simulink model "DCMotorSystem"  (R2018b)
settings: Solver=FixedStepAuto  StartTime=0.0  StopTime=50  FixedStep=10^-5  RelTol=1e-3
undefined symbols (not defined in the file or in its folder): Kd, Kp
settings Model: Creator=Seko  LastModifiedBy=Seko

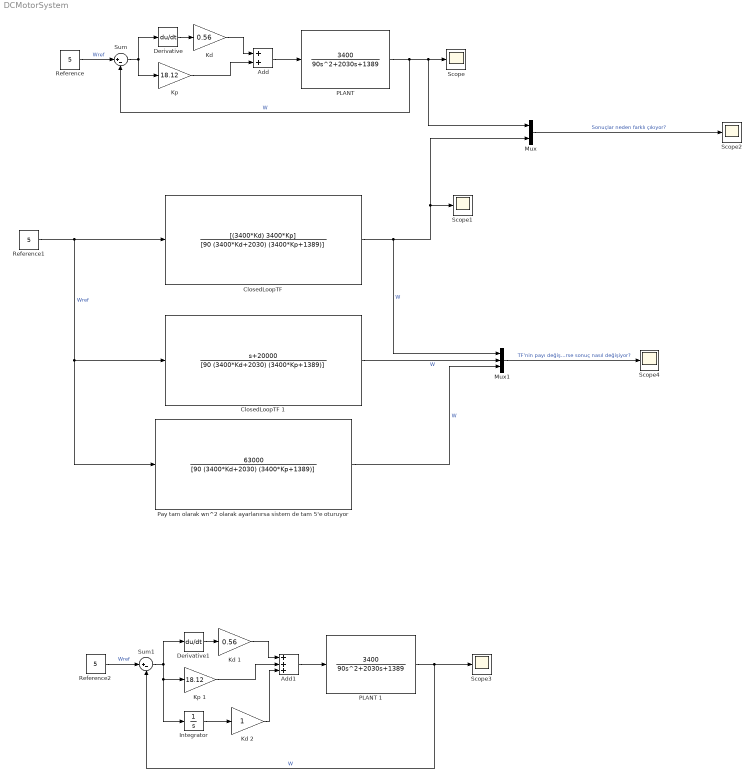
== system DCMotorSystem ==
  Add : Sum
  Add1 : Sum  Inputs=+++
  "ClosedLoopTF " : TransferFcn  Numerator=[(3400*Kd) 3400*Kp]  Denominator=[90 (3400*Kd+2030) (3400*Kp+1389)]
  ClosedLoopTF 1 : TransferFcn  Numerator=[1 20000]  Denominator=[90 (3400*Kd+2030) (3400*Kp+1389)]
  Derivative : Derivative
  Derivative1 : Derivative
  Integrator : Integrator
  "Kd " : Gain  Gain=0.56
  Kd 1 : Gain  Gain=0.56
  Kd 2 : Gain
  "Kp " : Gain  Gain=18.12
  Kp 1 : Gain  Gain=18.12
  Mux : Mux  Inputs=2
  Mux1 : Mux  Inputs=3
  "PLANT " : TransferFcn  Numerator=[3400]  Denominator=[90 2030 1389]
  PLANT 1 : TransferFcn  Numerator=[3400]  Denominator=[90 2030 1389]
  Pay tam olarak wn^2 olarak ayarlanırsa sistem de tam 5'e oturuyor : TransferFcn  Numerator=[63000]  Denominator=[90 (3400*Kd+2030) (3400*Kp+1389)]
  Reference : Constant  Value=5
  Reference1 : Constant  Value=5
  Reference2 : Constant  Value=5
  Scope{,1..4} (5 alike) : Scope
  Sum : Sum  Inputs=|+-
  Sum1 : Sum  Inputs=|+-
  wires:
  Reference/1 -> Sum/1  "Wref"
  "PLANT "/1 -> Sum/2, Mux/1, Scope/1  "W"
  "Kp "/1 -> Add/2
  Add/1 -> "PLANT "/1
  Derivative/1 -> "Kd "/1
  Sum/1 -> Derivative/1, "Kp "/1
  Reference1/1 -> Pay tam olarak wn^2 olarak ayarlanırsa sistem de tam 5'e oturuyor/1, ClosedLoopTF 1/1, "ClosedLoopTF "/1  "Wref"
  "ClosedLoopTF "/1 -> Mux1/1, Mux/2, Scope1/1  "W"
  "Kd "/1 -> Add/1
  Mux/1 -> Scope2/1  "Sonuçlar neden farklı çıkıyor?"
  Mux1/1 -> Scope4/1  "TF'nin payı değişirse sonuç nasıl değişiyor?"
  ClosedLoopTF 1/1 -> Mux1/2  "W"
  Pay tam olarak wn^2 olarak ayarlanırsa sistem de tam 5'e oturuyor/1 -> Mux1/3  "W"
  Kp 1/1 -> Add1/2
  Derivative1/1 -> Kd 1/1
  Add1/1 -> PLANT 1/1
  Reference2/1 -> Sum1/1  "Wref"
  Sum1/1 -> Derivative1/1, Integrator/1, Kp 1/1
  Kd 1/1 -> Add1/1
  PLANT 1/1 -> Sum1/2, Scope3/1  "W"
  Integrator/1 -> Kd 2/1
  Kd 2/1 -> Add1/3
